simulink model "CoupledTanks_Workspace"  (R2021a)
settings: Solver=ode4  StartTime=0.0  StopTime=inf  FixedStep=0.002  RelTol=1e-3  EnableMultiTasking=on
undefined symbols (not defined in the file or in its folder): DiscIntNeverNeededParam
libraries: quarc_library x7, simulink x4
settings Model: SimulationMode=external  ExtModeTrigDuration=10000  Creator=MLevis  LastModifiedBy=pmartin
settings SolverCC: AlgebraicLoopSolver=TrustRegion  PositivePriorityOrder=on
settings DataIOCC: LimitDataPoints=on  SaveFormat=Array  SignalLoggingSaveFormat=ModelDataLogs  ReturnWorkspaceOutputs=off
settings OptimizationCC: ExpressionDepthLimit=2147483647  InitFltsAndDblsToZero=on
settings DebuggingCC: SaveWithParameterizedLinksMsg=none  UnderspecifiedInitializationDetection=Classic  MergeDetectMultiDrivingBlocksExec=none  SolverPrmCheckMsg=warning  FcnCallInpInsideContextMsg=warning  AllowSymbolicDim=off  StateNameClashWarn=warning  SFUnexpectedBacktrackingDiag=warning  SFNoUnconditionalDefaultTransitionDiag=warning  SFExecutionAtInitializationDiag=none  SFMachineParentedDataDiag=warning  ArithmeticOperatorsInVariantConditions=warning
settings ModelReferenceCC: PropagateSignalLabelsOutOfModel=off
settings SFSimCC: SimUseLocalCustomCode=off  CustomCodeUndefinedFunction=UseInterfaceOnly
settings RTWCC: Description=QUARC Win64 Target Using Toolchain  SystemTargetFile=quarc_win64.tlc  TemplateMakefile=quarc_default_tmf  RTWUseLocalCustomCode=off  Toolchain=QUARC win64 | nmake (64-bit Windows)  BuildConfiguration=Faster Runs
settings CodeAppCC: StateflowObjectComments=on
settings STFCustomTargetCC: ConcurrentExecutionCompliant=on  SystemTargetFile=quarc_win64.tlc
settings GRTTargetCC: TargetLangStandard=C89/C90 (ANSI)  ParMdlRefBuildCompliant=off  CompOptLevelCompliant=off  CombineOutputUpdateFcns=off  MatFileLogging=off  CPPClassGenCompliant=off  GRTInterface=on  ExtMode=on  ExtModeMexFile=quarc_comm
settings ConfigComp: CovMetricSettings=dw  CovSaveCumulativeToWorkspaceVar=on  CovSaveSingleToWorkspaceVar=on  CovExternalEMLEnable=off

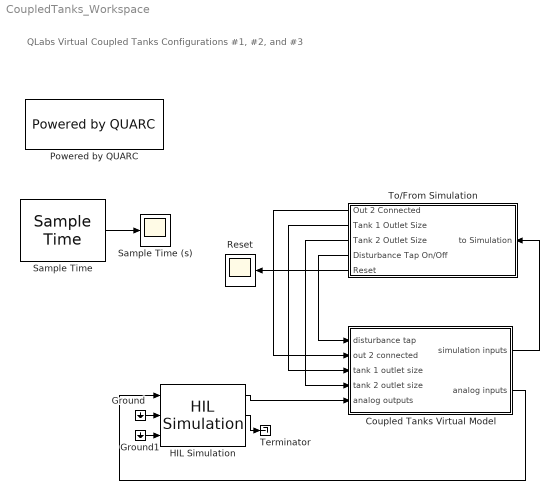
== system CoupledTanks_Workspace ==
  note: QLabs Virtual Coupled Tanks
      | Configurations #1, #2, and #3
  Coupled Tanks Virtual Model : Subsystem
  Ground : Ground
  Ground1 : Ground
  HIL Simulation : quarc_library/Data Acquisition/Generic/Configuration/HIL Simulation  uri=tcpip://localhost:18950  board_type=q8_usb  board_id=0  sample_time=qc_get_step_size  active=on  num_clocks=1  num_interrupts=0  num_analog_inputs=8  num_analog_outputs=8  initial_analog=[]  num_digital_io=0  num_digital_inputs=8  num_digital_outputs=8  initial_digital=[]  num_encoder_inputs=8  num_pwm_outputs=8  initial_pwm=[]  other_inputs=[]  other_outputs=[]  initial_other=[]  integer_properties=[]  double_properties=[]  string_properties=[]
      settings: SourceProductName=QUARC Targets
  Powered by QUARC : quarc_library/Logos/Powered by QUARC
  Reset : Scope
  Sample Time : quarc_library/Sources/Time/Sample Time  Priority=-99  sample_time=qc_get_step_size
  Sample Time (s) : Scope
  Terminator : Terminator
  To/From Simulation : Subsystem
  wires:
  HIL Simulation/1 -> Coupled Tanks Virtual Model/5(analog outputs)
  Ground/1 -> HIL Simulation/2
  Ground1/1 -> HIL Simulation/3
  HIL Simulation/2 -> Terminator/1
  Sample Time/1 -> Sample Time (s)/1
  To/From Simulation/3(Tank 2 Outlet Size) -> Coupled Tanks Virtual Model/4(tank 2 outlet size)
  To/From Simulation/2(Tank 1 Outlet Size) -> Coupled Tanks Virtual Model/3(tank 1 outlet size)
  To/From Simulation/4(Disturbance Tap On/Off) -> Coupled Tanks Virtual Model/1(disturbance tap)
  To/From Simulation/1(Out 2 Connected) -> Coupled Tanks Virtual Model/2(out 2 connected)
  Coupled Tanks Virtual Model/1(simulation inputs) -> To/From Simulation/1(to Simulation)
  Coupled Tanks Virtual Model/2(analog inputs) -> HIL Simulation/1
  To/From Simulation/5(Reset) -> Reset/1

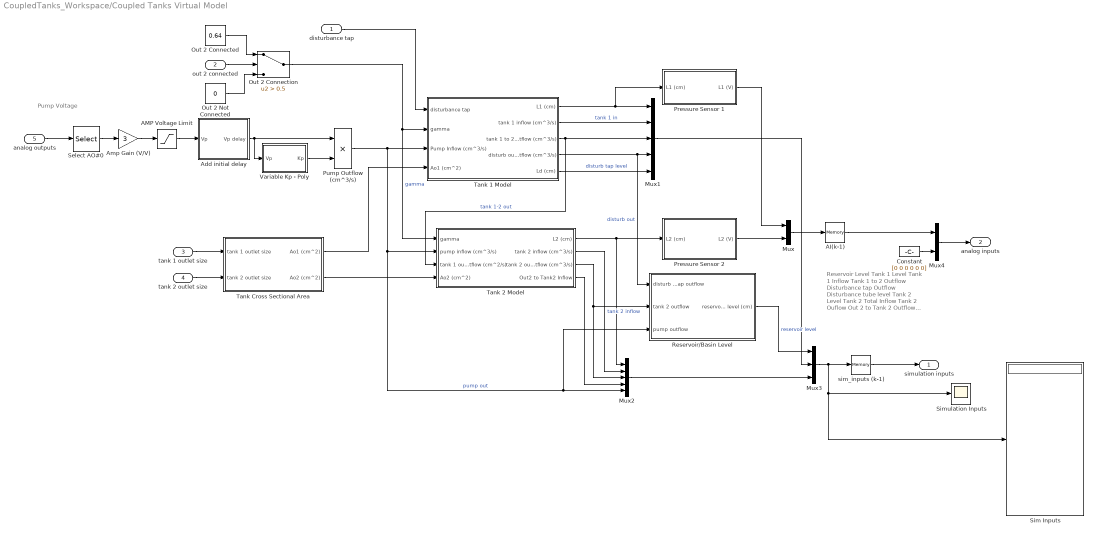
== system CoupledTanks_Workspace/Coupled Tanks Virtual Model ==
  note: Reservoir Level
      | Tank 1 Level
      | Tank 1 Inflow
      | Tank 1 to 2 Outflow
      | Disturbance tap Outflow
      | Disturbance tube level
      | Tank 2 Level
      | Tank 2 Total Inflow
      | Tank 2 Ouflow
      | Out 2 to Tank 2 Outflow
      | Pump Outflow
  note: Pump
      | Voltage
  disturbance tap : Inport
  out 2 connected : Inport  Port=2
  tank 1 outlet size : Inport  Port=3
  tank 2 outlet size : Inport  Port=4
  analog outputs : Inport  Port=5
  AI(k-1) : Memory
  AMP Voltage Limit : Saturate  UpperLimit=22  LowerLimit=0
  Add initial delay : Subsystem
  Amp Gain (V/V) : Gain  Gain=3
  Constant : Constant  Value=[0 0 0 0 0 0]
  Mux : Mux  Inputs=2
  Mux1 : Mux  Inputs=5
  Mux2 : Mux  Inputs=5
  Mux3 : Mux  Inputs=3
  Mux4 : Mux  Inputs=[2 6]
  Out 2 Connected : Constant  Value=0.64
  Out 2 Connection : Switch  Criteria=u2 > Threshold  Threshold=0.5
  Out 2 Not Connected : Constant  Value=0
  Pressure Sensor 1 : Subsystem
  Pressure Sensor 2 : Subsystem
  Pump Outflow (cm^3/s) : Product
  Reservoir/Basin Level : Subsystem
  Select AO#0 : Selector  InputPortWidth=8  IndexOptions=Index vector (dialog)  Indices=[1]  OutputSizes=1
  Sim Inputs : Display
      settings: Decimation=50
  Simulation Inputs : Scope
  Tank 1 Model : Subsystem
  Tank 2 Model : Subsystem
  Tank Cross Sectional Area : Subsystem
  Variable Kp - Poly : Subsystem
  sim_inputs (k-1) : Memory
  simulation inputs : Outport  VectorParamsAs1DForOutWhenUnconnected=off
  analog inputs : Outport  Port=2  InitialOutput=0  VectorParamsAs1DForOutWhenUnconnected=off
  wires:
  analog outputs/1 -> Select AO#0/1
  Mux/1 -> AI(k-1)/1
  out 2 connected/1 -> Out 2 Connection/2
  Out 2 Connected/1 -> Out 2 Connection/1
  Out 2 Not Connected/1 -> Out 2 Connection/3
  Out 2 Connection/1 -> Tank 2 Model/1(gamma), Tank 1 Model/2(gamma)  "gamma"
  Select AO#0/1 -> Amp Gain (V/V)/1
  Amp Gain (V/V)/1 -> AMP Voltage Limit/1
  AMP Voltage Limit/1 -> Add initial delay/1(Vp)
  Pump Outflow (cm^3/s)/1 -> Tank 2 Model/2(pump inflow (cm^3/s)), Reservoir/Basin Level/3(pump outflow), Mux2/5, Tank 1 Model/3(Pump Inflow (cm^3/s))  "pump out"
  Tank 1 Model/1(L1 (cm)) -> Mux1/1, Pressure Sensor 1/1(L1 (cm))
  tank 1 outlet size/1 -> Tank Cross Sectional Area/1(tank 1 outlet size)
  tank 2 outlet size/1 -> Tank Cross Sectional Area/2(tank 2 outlet size)
  Tank Cross Sectional Area/1(Ao1 (cm^2)) -> Tank 1 Model/4(Ao1 (cm^2))
  Tank 1 Model/3(tank 1 to 2 outflow (cm^3/s)) -> Tank 2 Model/3(tank 1 outflow (cm^2/s)), Mux1/3  "tank 1-2 out"
  Tank Cross Sectional Area/2(Ao2 (cm^2)) -> Tank 2 Model/4(Ao2 (cm^2))
  Tank 2 Model/2(tank 2 inflow (cm^3/s)) -> Mux2/2  "tank 2 inflow"
  Pressure Sensor 1/1(L1 (V)) -> Mux/1
  Tank 2 Model/1(L2 (cm)) -> Mux2/1, Pressure Sensor 2/1(L2 (cm))
  Pressure Sensor 2/1(L2 (V)) -> Mux/2
  sim_inputs (k-1)/1 -> simulation inputs/1
  Tank 1 Model/2(tank 1 inflow (cm^3/s)) -> Mux1/2  "tank 1 in"
  Mux2/1 -> Mux3/3
  Mux1/1 -> Mux3/2
  Mux3/1 -> sim_inputs (k-1)/1, Sim Inputs/1, Simulation Inputs/1
  Tank 2 Model/3(tank 2 outflow (cm^3/s)) -> Mux2/3, Reservoir/Basin Level/2(tank 2 outflow)
  Reservoir/Basin Level/1(reservoir level (cm)) -> Mux3/1  "reservoir level"
  Tank 1 Model/4(disturb outflow (cm^3/s)) -> Reservoir/Basin Level/1(disturb tap outflow), Mux1/4  "disturb out"
  disturbance tap/1 -> Tank 1 Model/1(disturbance tap)
  Tank 1 Model/5(Ld (cm)) -> Mux1/5  "disturb tap level"
  Add initial delay/1(Vp delay) -> Variable Kp - Poly/1(Vp), Pump Outflow (cm^3/s)/1
  Variable Kp - Poly/1(Kp) -> Pump Outflow (cm^3/s)/2
  AI(k-1)/1 -> Mux4/1
  Mux4/1 -> analog inputs/1
  Constant/1 -> Mux4/2
  Tank 2 Model/4(Out2 to Tank2 Inflow) -> Mux2/4

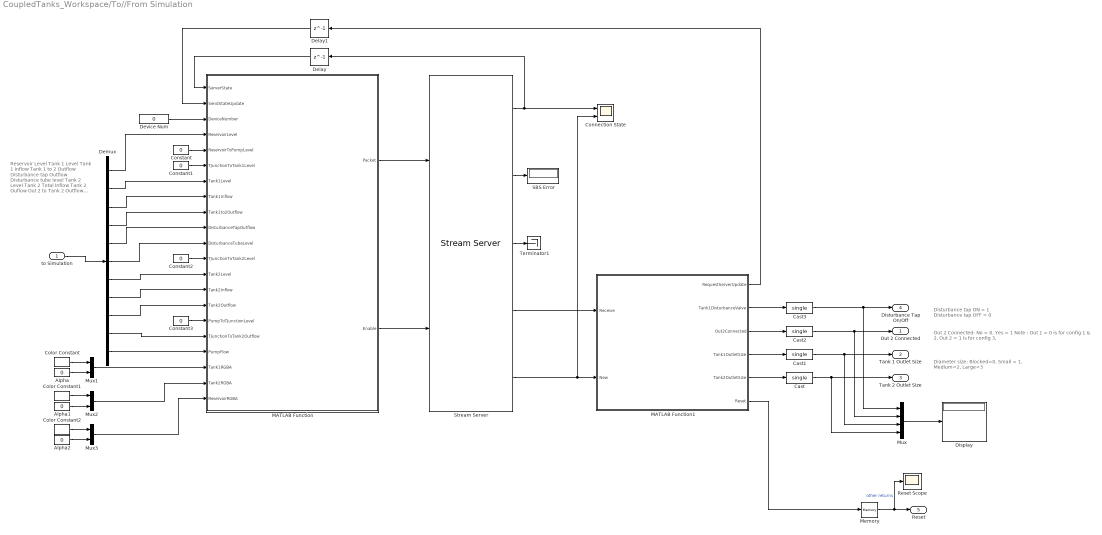
== system CoupledTanks_Workspace/To//From Simulation ==
  note: Disturbance tap ON = 1
      | Disturbance tap OFF = 0
  note: Diameter size:
      | Blocked=0, Small = 1, Medium=2, Large=3
  note: Out 2 Connected:
      | No = 0, Yes = 1
      | Note : Out 1 = 0 is for config 1 & 2, Out 2 = 1 is for config 3,
  note: Reservoir Level
      | Tank 1 Level
      | Tank 1 Inflow
      | Tank 1 to 2 Outflow
      | Disturbance tap Outflow
      | Disturbance tube level
      | Tank 2 Level
      | Tank 2 Total Inflow
      | Tank 2 Ouflow
      | Out 2 to Tank 2 Outflow
      | Pump Outflow
  to Simulation : Inport
  Alpha : Constant  Value=0
  Alpha1 : Constant  Value=0
  Alpha2 : Constant  Value=0
  Cast{,1..3} (4 alike) : DataTypeConversion  OutDataTypeStr=single
  Color Constant : quarc_library/Sources/Signals/Color Constant  color=[0.8902 0.1059 0.1373]
      settings: SourceProductName=QUARC Targets
  Color Constant1 : quarc_library/Sources/Signals/Color Constant  color=[0.8902 0.1059 0.1373]
      settings: SourceProductName=QUARC Targets
  Color Constant2 : quarc_library/Sources/Signals/Color Constant  color=[0.8902 0.1059 0.1373]
      settings: SourceProductName=QUARC Targets
  "Connection State " : Scope  NumInputPorts=2
  Constant{,1..3} (4 alike) : Constant  Value=0
  Delay : Delay  DelayLength=1
  Delay1 : Delay  DelayLength=1
  Demux : Demux  Outputs=[1 1 1 1 1 1 1 1 1 1 1]
  Device Num : Constant  Value=0
  Display : Display
  MATLAB Function : MATLAB Function  TreatAsAtomicUnit=on
  MATLAB Function1 : MATLAB Function  TreatAsAtomicUnit=on
  Memory : Memory
  Mux : Mux
  Mux1 : Mux  Inputs=2
  Mux2 : Mux  Inputs=2
  Mux3 : Mux  Inputs=2
  "Reset Scope " : Scope
  SBS Error : Display
  Stream Server : quarc_library/Communications/Basic/Stream Server  uri_source=Specify via dialog (do not evaluate)  uri=tcpip://remotehost:18001?nagle='off'  apply_uri_to_all_configs=on  send_buffer_size=65537  receive_buffer_size=65537  byte_order=little endian (Intel - LSB first)  optimization=Minimum latency  send_options=Send all data  receive_options=Receive all data  default_value=[0]  sample_time=qc_get_step_size  active=on  implementation=Use blocking I/O in a separate thread  send_fifo_size=3  receive_fifo_size=3  send_priority=0  receive_priority=0  send_dimensions=on  receive_dimensions=on  max_dimensions=65537  data_type=uint8  type_expr=BusObject
      settings: AttributesFormatString="\"tcpip://remotehost:18001?nagle='off'\""
  Terminator1 : Terminator
  Out 2 Connected : Outport  VectorParamsAs1DForOutWhenUnconnected=off
  Tank 1 Outlet Size : Outport  Port=2  VectorParamsAs1DForOutWhenUnconnected=off
  Tank 2 Outlet Size : Outport  Port=3  VectorParamsAs1DForOutWhenUnconnected=off
  Disturbance Tap On/Off : Outport  Port=4  VectorParamsAs1DForOutWhenUnconnected=off
  Reset : Outport  Port=5  VectorParamsAs1DForOutWhenUnconnected=off
  wires:
  Stream Server/3 -> Terminator1/1
  Delay/1 -> MATLAB Function/1(ServerState)
  Stream Server/2 -> SBS Error/1
  to Simulation/1 -> Demux/1
  MATLAB Function1/6(Reset) -> Memory/1
  Delay1/1 -> MATLAB Function/2(SendStateUpdate)
  Memory/1 -> "Reset Scope "/1, Reset/1  "other returns"
  Stream Server/4 -> MATLAB Function1/1(Receive)
  Mux/1 -> Display/1
  MATLAB Function/2(Enable) -> Stream Server/2
  Stream Server/5 -> "Connection State "/2, MATLAB Function1/2(New)
  Device Num/1 -> MATLAB Function/3(DeviceNumber)
  Stream Server/1 -> Delay/1, "Connection State "/1
  MATLAB Function1/1(RequestServerUpdate) -> Delay1/1
  MATLAB Function/1(Packet) -> Stream Server/1
  Demux/1 -> MATLAB Function/4(ReservoirLevel)
  Constant/1 -> MATLAB Function/5(ReservoirToPumpLevel)
  Constant1/1 -> MATLAB Function/6(TJunctionToTank1Level)
  Constant2/1 -> MATLAB Function/12(TJunctionToTank2Level)
  Color Constant/1 -> Mux1/1
  Alpha/1 -> Mux1/2
  Alpha1/1 -> Mux2/2
  Color Constant1/1 -> Mux2/1
  Alpha2/1 -> Mux3/2
  Color Constant2/1 -> Mux3/1
  Mux1/1 -> MATLAB Function/19(Tank1RGBA)
  Mux2/1 -> MATLAB Function/20(Tank2RGBA)
  Mux3/1 -> MATLAB Function/21(ReservoirRGBA)
  Demux/9 -> MATLAB Function/15(Tank2Outflow)
  Demux/8 -> MATLAB Function/14(Tank2Inflow)
  Demux/7 -> MATLAB Function/13(Tank2Level)
  Demux/6 -> MATLAB Function/11(DisturbanceTubeLevel)
  Demux/5 -> MATLAB Function/10(DisturbanceTapOutflow)
  Demux/4 -> MATLAB Function/9(Tank1to2Outflow)
  Demux/3 -> MATLAB Function/8(Tank1Inflow)
  Demux/2 -> MATLAB Function/7(Tank1Level)
  Constant3/1 -> MATLAB Function/16(PumpToTJunctionLevel)
  MATLAB Function1/2(Tank1DisturbanceValve) -> Cast3/1
  MATLAB Function1/3(Out2Connected) -> Cast2/1
  Cast/1 -> Tank 2 Outlet Size/1, Mux/4
  Cast1/1 -> Tank 1 Outlet Size/1, Mux/3
  Cast2/1 -> Out 2 Connected/1, Mux/2
  Cast3/1 -> Disturbance Tap On/Off/1, Mux/1
  MATLAB Function1/4(Tank1OutletSize) -> Cast1/1
  MATLAB Function1/5(Tank2OutletSize) -> Cast/1
  Demux/11 -> MATLAB Function/18(PumpFlow)
  Demux/10 -> MATLAB Function/17(TJunctionToTank2Outflow)

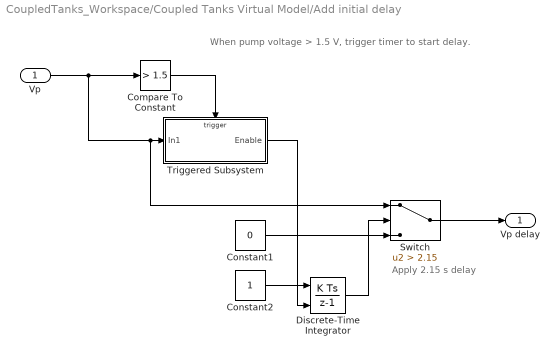
== system CoupledTanks_Workspace/Coupled Tanks Virtual Model/Add initial delay ==
  note: When pump voltage > 1.5 V, trigger timer to start delay.
  note: Apply 2.15 s delay
  Vp : Inport
  Compare To Constant : simulink/Logic and Bit Operations/Compare To Constant  relop=>  const=1.5  OutDataTypeStr=boolean
  Constant1 : Constant  Value=0
  Constant2 : Constant
  Discrete-Time Integrator : DiscreteIntegrator  ExternalReset=rising  SampleTime=-1  ICPrevOutput=DiscIntNeverNeededParam  ICPrevScaledInput=DiscIntNeverNeededParam
  Switch : Switch  Criteria=u2 > Threshold  Threshold=2.15
  Triggered Subsystem : Subsystem  TreatAsAtomicUnit=on
  Vp delay : Outport  VectorParamsAs1DForOutWhenUnconnected=off
  wires:
  Constant2/1 -> Discrete-Time Integrator/1
  Triggered Subsystem/1(Enable) -> Discrete-Time Integrator/2
  Vp/1 -> Compare To Constant/1, Switch/1, Triggered Subsystem/1(In1)
  Constant1/1 -> Switch/3
  Compare To Constant/1 -> Triggered Subsystem/Trigger
  Discrete-Time Integrator/1 -> Switch/2
  Switch/1 -> Vp delay/1

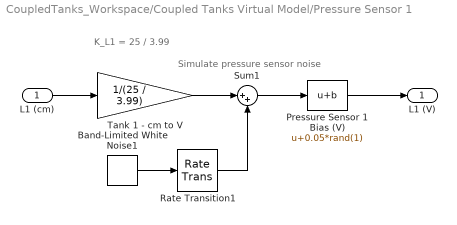
== system CoupledTanks_Workspace/Coupled Tanks Virtual Model/Pressure Sensor 1 ==
  note: K_L1 = 25 / 3.99
  note: Simulate pressure sensor noise
  L1 (cm) : Inport
  Band-Limited White Noise1 : simulink/Sources/Band-Limited White Noise  Cov=[3e-7]  Ts=0.01  seed=[23341]
  Pressure Sensor 1 Bias (V) : Bias  Bias=0.05*rand(1)
  Rate Transition1 : RateTransition
  Sum1 : Sum  Inputs=|++
  Tank 1 - cm to V : Gain  Gain=1/(25 / 3.99)
  L1 (V) : Outport  VectorParamsAs1DForOutWhenUnconnected=off
  wires:
  Rate Transition1/1 -> Sum1/2
  L1 (cm)/1 -> Tank 1 - cm to V/1
  Tank 1 - cm to V/1 -> Sum1/1
  Band-Limited White Noise1/1 -> Rate Transition1/1
  Pressure Sensor 1 Bias (V)/1 -> L1 (V)/1
  Sum1/1 -> Pressure Sensor 1 Bias (V)/1

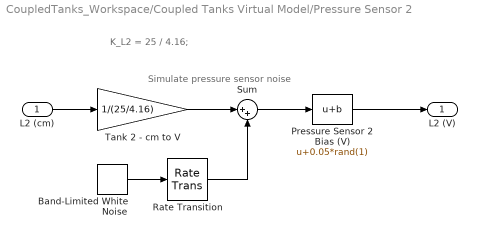
== system CoupledTanks_Workspace/Coupled Tanks Virtual Model/Pressure Sensor 2 ==
  note: K_L2 = 25 / 4.16;
  note: Simulate pressure sensor noise
  L2 (cm) : Inport
  Band-Limited White Noise : simulink/Sources/Band-Limited White Noise  Cov=[1.25e-5]  Ts=0.01  seed=[23341]
  Pressure Sensor 2 Bias (V) : Bias  Bias=0.05*rand(1)
  Rate Transition : RateTransition
  Sum : Sum  Inputs=|++
  Tank 2 - cm to V : Gain  Gain=1/(25/4.16)
  L2 (V) : Outport  VectorParamsAs1DForOutWhenUnconnected=off
  wires:
  Band-Limited White Noise/1 -> Rate Transition/1
  Rate Transition/1 -> Sum/2
  Sum/1 -> Pressure Sensor 2 Bias (V)/1
  Tank 2 - cm to V/1 -> Sum/1
  Pressure Sensor 2 Bias (V)/1 -> L2 (V)/1
  L2 (cm)/1 -> Tank 2 - cm to V/1

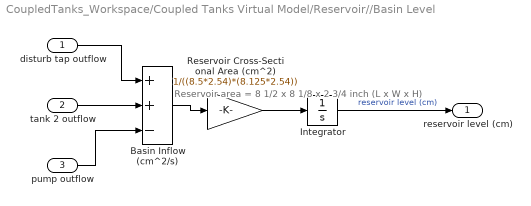
== system CoupledTanks_Workspace/Coupled Tanks Virtual Model/Reservoir//Basin Level ==
  note: Reservoir area = 8 1/2 x 8 1/8 x 2 3/4 inch (L x W x H)
  disturb tap outflow : Inport
  tank 2 outflow : Inport  Port=2
  pump outflow : Inport  Port=3
  Basin Inflow (cm^2/s) : Sum  Inputs=++-
  Integrator : Integrator  InitialCondition=2.54*1.75  LimitOutput=on  UpperSaturationLimit=2.54*2.75  LowerSaturationLimit=0
  Reservoir Cross-Sectional Area (cm^2) : Gain  Gain=1/((8.5*2.54)*(8.125*2.54))  SaturateOnIntegerOverflow=on  OutDataTypeStr=Inherit: Same as input  ParamDataTypeStr=Inherit: Same as input
  reservoir level (cm) : Outport  VectorParamsAs1DForOutWhenUnconnected=off
  wires:
  Reservoir Cross-Sectional Area (cm^2)/1 -> Integrator/1
  tank 2 outflow/1 -> Basin Inflow (cm^2/s)/2
  Integrator/1 -> reservoir level (cm)/1  "reservoir level (cm)"
  Basin Inflow (cm^2/s)/1 -> Reservoir Cross-Sectional Area (cm^2)/1
  disturb tap outflow/1 -> Basin Inflow (cm^2/s)/1
  pump outflow/1 -> Basin Inflow (cm^2/s)/3

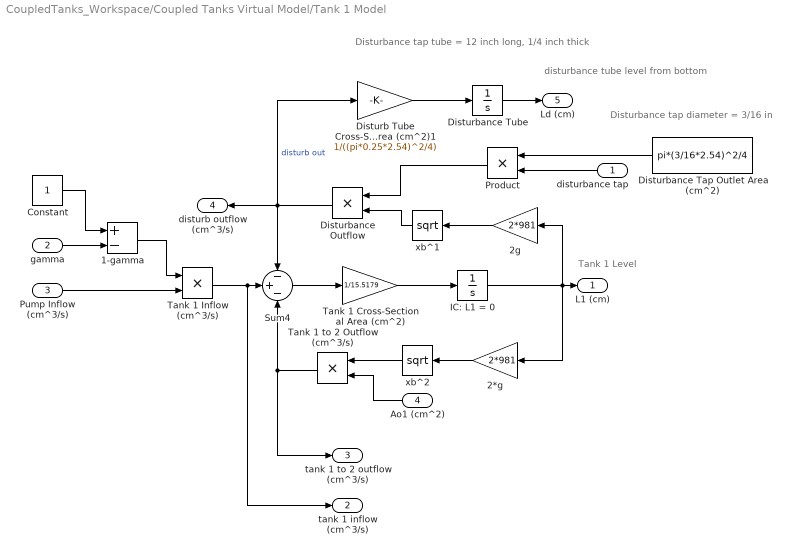
== system CoupledTanks_Workspace/Coupled Tanks Virtual Model/Tank 1 Model ==
  note: disturbance tube level from bottom
  note: Disturbance tap tube = 12 inch long, 1/4 inch thick
  note: Tank 1 Level
  note: Disturbance tap diameter = 3/16 in
  disturbance tap : Inport
  gamma : Inport  Port=2
  Pump Inflow (cm^3/s) : Inport  Port=3
  Ao1 (cm^2) : Inport  Port=4
  1-gamma : Sum  Inputs=+-
  2*g : Gain  Gain=2*981  SaturateOnIntegerOverflow=on  OutDataTypeStr=Inherit: Same as input  ParamDataTypeStr=Inherit: Same as input
  2g : Gain  Gain=2*981  SaturateOnIntegerOverflow=on  OutDataTypeStr=Inherit: Same as input  ParamDataTypeStr=Inherit: Same as input
  Constant : Constant
  Disturb Tube Cross-Sectional Area (cm^2)1 : Gain  Gain=1/((pi*0.25*2.54)^2/4)  SaturateOnIntegerOverflow=on  OutDataTypeStr=Inherit: Same as input  ParamDataTypeStr=Inherit: Same as input
  Disturbance Outflow : Product
  Disturbance Tap Outlet Area (cm^2) : Constant  Value=pi*(3/16*2.54)^2/4
  Disturbance Tube : Integrator  LimitOutput=on  UpperSaturationLimit=12*2.54  LowerSaturationLimit=0
  IC: L1 = 0 : Integrator  LimitOutput=on  UpperSaturationLimit=30  LowerSaturationLimit=0
  Product : Product
  Sum4 : Sum  Inputs=-+-  InputSameDT=on  SaturateOnIntegerOverflow=on  OutDataTypeStr=Inherit: Same as first input
  Tank 1 Cross-Sectional Area (cm^2) : Gain  Gain=1/15.5179  SaturateOnIntegerOverflow=on  OutDataTypeStr=Inherit: Same as input  ParamDataTypeStr=Inherit: Same as input
  Tank 1 Inflow (cm^3/s) : Product
  Tank 1 to 2 Outflow (cm^3/s) : Product
  xb^1 : Math  Operator=sqrt  SignedPower=on  SaturateOnIntegerOverflow=on
  xb^2 : Math  Operator=sqrt  SignedPower=on  SaturateOnIntegerOverflow=on
  L1 (cm) : Outport  VectorParamsAs1DForOutWhenUnconnected=off
  tank 1 inflow (cm^3/s) : Outport  Port=2  VectorParamsAs1DForOutWhenUnconnected=off
  tank 1 to 2 outflow (cm^3/s) : Outport  Port=3  VectorParamsAs1DForOutWhenUnconnected=off
  disturb outflow (cm^3/s) : Outport  Port=4  VectorParamsAs1DForOutWhenUnconnected=off
  Ld (cm) : Outport  Port=5  VectorParamsAs1DForOutWhenUnconnected=off
  wires:
  Pump Inflow (cm^3/s)/1 -> Tank 1 Inflow (cm^3/s)/2
  Tank 1 Cross-Sectional Area (cm^2)/1 -> IC: L1 = 0/1
  Ao1 (cm^2)/1 -> Tank 1 to 2 Outflow (cm^3/s)/2
  Sum4/1 -> Tank 1 Cross-Sectional Area (cm^2)/1
  IC: L1 = 0/1 -> 2g/1, 2*g/1, L1 (cm)/1
  Constant/1 -> 1-gamma/1
  1-gamma/1 -> Tank 1 Inflow (cm^3/s)/1
  2*g/1 -> xb^2/1
  gamma/1 -> 1-gamma/2
  Tank 1 to 2 Outflow (cm^3/s)/1 -> tank 1 to 2 outflow (cm^3/s)/1, Sum4/3
  xb^2/1 -> Tank 1 to 2 Outflow (cm^3/s)/1
  Tank 1 Inflow (cm^3/s)/1 -> tank 1 inflow (cm^3/s)/1, Sum4/2
  Product/1 -> Disturbance Outflow/1
  Disturbance Tap Outlet Area (cm^2)/1 -> Product/1
  disturbance tap/1 -> Product/2
  Disturbance Outflow/1 -> Disturb Tube Cross-Sectional Area (cm^2)1/1, disturb outflow (cm^3/s)/1, Sum4/1  "disturb out"
  2g/1 -> xb^1/1
  xb^1/1 -> Disturbance Outflow/2
  Disturb Tube Cross-Sectional Area (cm^2)1/1 -> Disturbance Tube/1
  Disturbance Tube/1 -> Ld (cm)/1

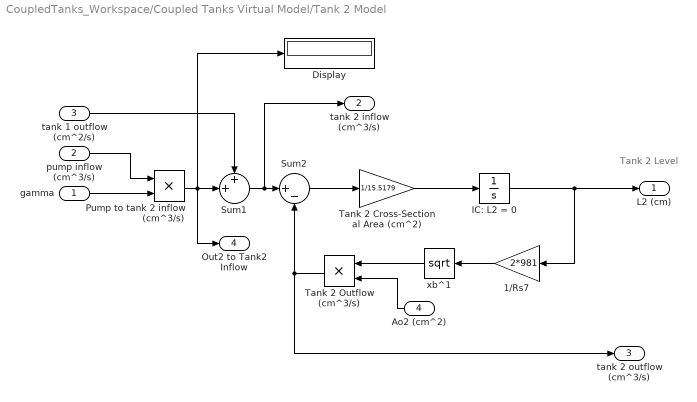
== system CoupledTanks_Workspace/Coupled Tanks Virtual Model/Tank 2 Model ==
  note: Tank 2 Level
  gamma : Inport
  pump inflow (cm^3/s) : Inport  Port=2
  tank 1 outflow (cm^2/s) : Inport  Port=3
  Ao2 (cm^2) : Inport  Port=4
  1/Rs7 : Gain  Gain=2*981  SaturateOnIntegerOverflow=on  OutDataTypeStr=Inherit: Same as input  ParamDataTypeStr=Inherit: Same as input
  Display : Display
      settings: Decimation=50
  IC: L2 = 0 : Integrator  LimitOutput=on  UpperSaturationLimit=30  LowerSaturationLimit=0
  Pump to tank 2 inflow (cm^3/s) : Product
  Sum1 : Sum  Inputs=++|  InputSameDT=on  SaturateOnIntegerOverflow=on  OutDataTypeStr=Inherit: Same as first input
  Sum2 : Sum  Inputs=|+-  InputSameDT=on  SaturateOnIntegerOverflow=on  OutDataTypeStr=Inherit: Same as first input
  Tank 2 Cross-Sectional Area (cm^2) : Gain  Gain=1/15.5179  SaturateOnIntegerOverflow=on  OutDataTypeStr=Inherit: Same as input  ParamDataTypeStr=Inherit: Same as input
  Tank 2 Outflow (cm^3/s) : Product
  xb^1 : Math  Operator=sqrt  SignedPower=on  SaturateOnIntegerOverflow=on
  L2 (cm) : Outport  VectorParamsAs1DForOutWhenUnconnected=off
  tank 2 inflow (cm^3/s) : Outport  Port=2  VectorParamsAs1DForOutWhenUnconnected=off
  tank 2 outflow (cm^3/s) : Outport  Port=3  VectorParamsAs1DForOutWhenUnconnected=off
  Out2 to Tank2 Inflow : Outport  Port=4  VectorParamsAs1DForOutWhenUnconnected=off
  wires:
  Tank 2 Outflow (cm^3/s)/1 -> Sum2/2, tank 2 outflow (cm^3/s)/1
  pump inflow (cm^3/s)/1 -> Pump to tank 2 inflow (cm^3/s)/1
  gamma/1 -> Pump to tank 2 inflow (cm^3/s)/2
  xb^1/1 -> Tank 2 Outflow (cm^3/s)/1
  Tank 2 Cross-Sectional Area (cm^2)/1 -> IC: L2 = 0/1
  Sum2/1 -> Tank 2 Cross-Sectional Area (cm^2)/1
  1/Rs7/1 -> xb^1/1
  IC: L2 = 0/1 -> L2 (cm)/1, 1/Rs7/1
  Ao2 (cm^2)/1 -> Tank 2 Outflow (cm^3/s)/2
  Sum1/1 -> tank 2 inflow (cm^3/s)/1, Sum2/1
  Pump to tank 2 inflow (cm^3/s)/1 -> Display/1, Out2 to Tank2 Inflow/1, Sum1/2
  tank 1 outflow (cm^2/s)/1 -> Sum1/1

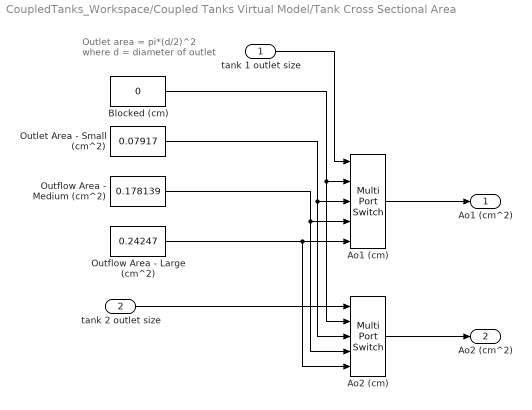
== system CoupledTanks_Workspace/Coupled Tanks Virtual Model/Tank Cross Sectional Area ==
  note: Outlet area = pi*(d/2)^2
      | where d = diameter of outlet
  tank 1 outlet size : Inport
  tank 2 outlet size : Inport  Port=2
  Ao1 (cm) : MultiPortSwitch  DataPortOrder=Zero-based contiguous  Inputs=4  zeroidx=on
  Ao2 (cm) : MultiPortSwitch  DataPortOrder=Zero-based contiguous  Inputs=4  zeroidx=on
  Blocked (cm) : Constant  Value=0
  Outflow Area - Large (cm^2) : Constant  Value=0.24247
  Outflow Area - Medium (cm^2) : Constant  Value=0.178139
  Outlet Area - Small (cm^2) : Constant  Value=0.07917
  Ao1 (cm^2) : Outport  VectorParamsAs1DForOutWhenUnconnected=off
  Ao2 (cm^2) : Outport  Port=2  VectorParamsAs1DForOutWhenUnconnected=off
  wires:
  tank 1 outlet size/1 -> Ao1 (cm)/1
  Outlet Area - Small (cm^2)/1 -> Ao2 (cm)/3, Ao1 (cm)/3
  tank 2 outlet size/1 -> Ao2 (cm)/1
  Ao1 (cm)/1 -> Ao1 (cm^2)/1
  Outflow Area - Large (cm^2)/1 -> Ao2 (cm)/5, Ao1 (cm)/5
  Outflow Area - Medium (cm^2)/1 -> Ao2 (cm)/4, Ao1 (cm)/4
  Ao2 (cm)/1 -> Ao2 (cm^2)/1
  Blocked (cm)/1 -> Ao2 (cm)/2, Ao1 (cm)/2

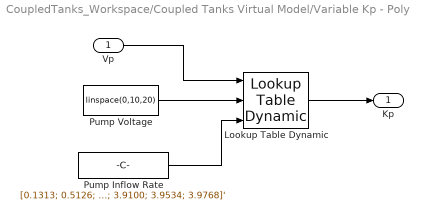
== system CoupledTanks_Workspace/Coupled Tanks Virtual Model/Variable Kp - Poly ==
  Vp : Inport
  Lookup Table Dynamic : simulink/Lookup Tables/Lookup Table Dynamic  LookUpMeth=Interpolation-Use End Values  OutDataType=fixdt('double')  OutScaling=[]  OutputDataTypeScalingMode=Specify via dialog  OutDataTypeStr=double  DoSatur=off
  Pump Inflow Rate : Constant  Value=[0.1313; 0.5126; 0.8741; 1.2156; 1.5373; 1.8391; 2.1211; 2.3831; 2.6253; 2.8476; 3.0500; 3.2325;3.3951;3.5379;3.6607; 3.7637; 3.8468; 3.9100; 3.9534; 3.9768]'
  Pump Voltage : Constant  Value=linspace(0,10,20)
  Kp : Outport  VectorParamsAs1DForOutWhenUnconnected=off
  wires:
  Pump Voltage/1 -> Lookup Table Dynamic/2
  Lookup Table Dynamic/1 -> Kp/1
  Pump Inflow Rate/1 -> Lookup Table Dynamic/3
  Vp/1 -> Lookup Table Dynamic/1

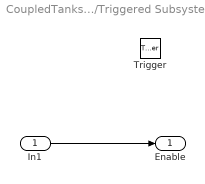
== system CoupledTanks_Workspace/Coupled Tanks Virtual Model/Add initial delay/Triggered Subsystem ==
  In1 : Inport
  Trigger : TriggerPort  VariantControl=Variant
  Enable : Outport  VectorParamsAs1DForOutWhenUnconnected=off
  wires:
  In1/1 -> Enable/1

== matlab function CoupledTanks_Workspace/To//From Simulation/MATLAB Function1 ==
  data: Receive input size=65537; RequestServerUpdate output; New input; Tank1DisturbanceValve output; Out2Connected output; Tank1OutletSize output; Tank2OutletSize output; Reset output
function [RequestServerUpdate, Tank1DisturbanceValve, Out2Connected, Tank1OutletSize, Tank2OutletSize, Reset]  = CoupledTanksDecodePacket(Receive, New)

%% Setup

persistent iTank1DisturbanceValve;
persistent iOut2Connected;
persistent iTank1OutletSize;
persistent iTank2OutletSize;

if isempty(iTank1DisturbanceValve)
    iTank1DisturbanceValve = single(0);
    iOut2Connected = uint8(0);
    iTank1OutletSize = uint8(0);
    iTank2OutletSize = uint8(0);
end

% Need to assign outputs here even though they are reassigned at the end
% since matlab can't determine the signal widths
Tank1DisturbanceValve = single(0);
Out2Connected = uint8(0);
Tank1OutletSize = uint8(0);
Tank2OutletSize = uint8(0);
Reset = 0;

RequestServerUpdate = 0;
PacketSize = length(Receive);

% Packet > 0, new data, and magic number in first index
if ((PacketSize > 0) && (New == 1) && (Receive(1) == uint8(123)))
    
    %skip magic number
    Index = int32(2);
    
    while(Index <= PacketSize)
       
        %% Get container details
        ContainerSize = typecast(uint8(flip(Receive(Index:Index+3))), 'int32');
        DeviceID = typecast(uint8(flip(Receive(Index+4:Index+7))), 'int32');
        DeviceNum = typecast(uint8(flip(Receive(Index+8:Index+11))), 'int32');
        DeviceFunction = uint8(Receive(Index+12));
        PayloadStart = Index+13;
        PayloadEnd = Index+ContainerSize-1;
        
        %% Pass container to appropriate decoding function
        if (DeviceID == 30) %is this an Coupled Tank container?
            
            if (DeviceFunction == 11) %UE4 State Response
                [iTank1DisturbanceValve] = CoupledTanksDecodeUE4StateContainer(Receive, PayloadStart);
                RequestServerUpdate = 1;
            elseif (DeviceFunction == 13) %Mode change
                [iOut2Connected, iTank1OutletSize, iTank2OutletSize] = CoupledTanksDecodeModeContainer(Receive, PayloadStart);  
            end
        
        elseif (DeviceID == 1001) %Simulink notification
            if (DeviceFunction == 200) %Reset button
                Reset = 1;
            end
        end
        
        
        
        %% Process next container if any data is left.
        Index = Index+ContainerSize;
    end


end

Tank1DisturbanceValve = iTank1DisturbanceValve;
Out2Connected = iOut2Connected;
Tank1OutletSize = iTank1OutletSize;
Tank2OutletSize = iTank2OutletSize;

== matlab function CoupledTanks_Workspace/To//From Simulation/MATLAB Function ==
  settings: updateMethod=DISCRETE  sampleTime=qc_get_step_size
  data: Packet output size=65537; ServerState input; SendStateUpdate input; Enable output; DeviceNumber input; ReservoirLevel input; ReservoirToPumpLevel input; TJunctionToTank1Level input; Tank1Level input; Tank1Inflow input; Tank1to2Outflow input; DisturbanceTapOutflow input; DisturbanceTubeLevel input; TJunctionToTank2Level input; Tank2Level input; Tank2Inflow input; Tank2Outflow input; PumpToTJunctionLevel input; TJunctionToTank2Outflow input; PumpFlow input; Tank1RGBA input; Tank2RGBA input; ReservoirRGBA input
function [Packet,Enable] = CoupledTanksMakePacket(ServerState, SendStateUpdate, DeviceNumber, ReservoirLevel, ReservoirToPumpLevel, TJunctionToTank1Level, Tank1Level, Tank1Inflow, Tank1to2Outflow, DisturbanceTapOutflow, DisturbanceTubeLevel, TJunctionToTank2Level, Tank2Level, Tank2Inflow, Tank2Outflow, PumpToTJunctionLevel, TJunctionToTank2Outflow, PumpFlow, Tank1RGBA, Tank2RGBA, ReservoirRGBA) 

% Be sure to set the maximum signal size of the variable size Packet port 
% in Simulink->Edit Data of the editor window.  Size should be 65537 or
% larger to ensure that the stream server generates a 4 byte packet size.

%% Setup
persistent LastServerState;

if isempty(LastServerState)
    LastServerState = uint8(0);
end

Enable = 0;
Packet = uint8([]);

%% On connection
if ((ServerState == 2) && (LastServerState ~= 2))
    Packet = CoupledTanksMakeCommandStateContainer(DeviceNumber, ReservoirLevel, ReservoirToPumpLevel, TJunctionToTank1Level, Tank1Level, Tank1Inflow, Tank1to2Outflow, DisturbanceTapOutflow, DisturbanceTubeLevel, TJunctionToTank2Level, TJunctionToTank2Outflow, Tank2Level, Tank2Inflow, Tank2Outflow, PumpToTJunctionLevel, PumpFlow, Tank1RGBA, Tank2RGBA, ReservoirRGBA);
    Packet = [Packet; CoupledTanksMakeModeRequestContainer(DeviceNumber)];
end

%% Send new State Container
% Previous state processed, send a new one
if (SendStateUpdate)
    Packet = CoupledTanksMakeCommandStateContainer(DeviceNumber, ReservoirLevel, ReservoirToPumpLevel, TJunctionToTank1Level, Tank1Level, Tank1Inflow, Tank1to2Outflow, DisturbanceTapOutflow, DisturbanceTubeLevel, TJunctionToTank2Level, TJunctionToTank2Outflow, Tank2Level, Tank2Inflow, Tank2Outflow, PumpToTJunctionLevel, PumpFlow, Tank1RGBA, Tank2RGBA, ReservoirRGBA);
   
end

%% Transmit
% If we have data to send, enable the transmit
PacketLength = length(Packet);

if (PacketLength > 0)
    % Add magic byte.  This is just for error handling and isn't typically
    % required in simulink, but useful in lower-level languages like Python
    Packet = [uint8(123); Packet];
    
    Enable = 1; 
end


LastServerState = ServerState;
